simulink model "sensorExpoler_Lab_13"  (R2026a)
settings: Solver=FixedStepDiscrete  StopTime=inf  FixedStep=0.001
undefined symbols (not defined in the file): Blocking, Non
libraries: simulink x2, amg_usbconverter_n_connect_lib x2
settings Model: Creator=pboon  LastModifiedBy=Lenovo

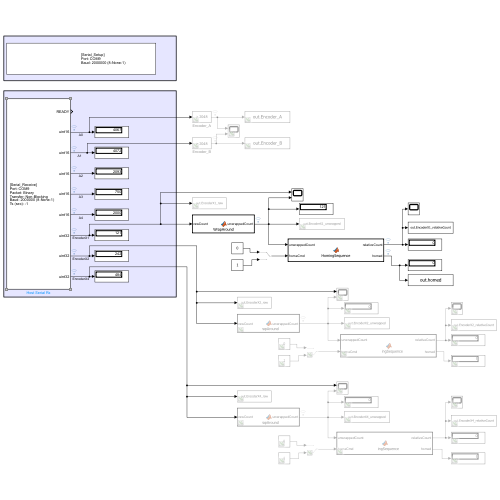
[thumbnail: Simulink's stored preview of the top-level diagram]
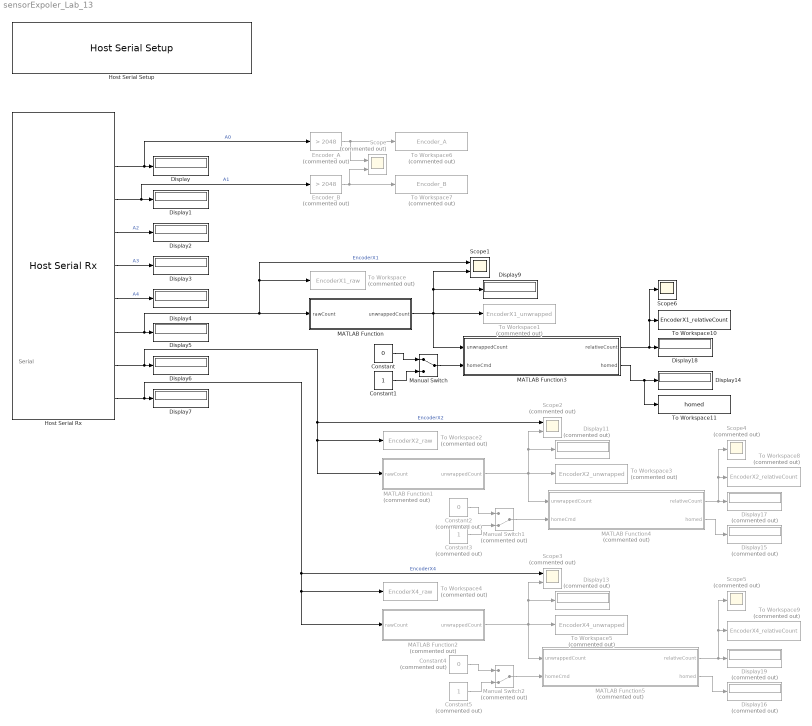
== system sensorExpoler_Lab_13 ==
  note: Serial
  Constant : Constant  Value=0
  Constant1 : Constant
  Constant2 : Constant  Commented=on  Value=0
  Constant3 : Constant  Commented=on
  Constant4 : Constant  Commented=on  Value=0
  Constant5 : Constant  Commented=on
  Display{,1..7,9,14,18} (11 alike) : Display
  Display{11,13,15..17,19} (6 alike) : Display  Commented=on
  Encoder_A : simulink/Logic and Bit Operations/Compare To Constant  Commented=on  relop=>  const=2048  OutDataTypeStr=boolean
  Encoder_B : simulink/Logic and Bit Operations/Compare To Constant  Commented=on  relop=>  const=2048  OutDataTypeStr=boolean
  Host Serial Rx : amg_usbconverter_n_connect_lib/Host Serial Rx  conf=rx  port=COM9  baudrate=2000000  databits=8  parity=None  stopbit=1  flowcontrol=None  transfer=Non-Blocking  timeout=5  packetmode=Binary  enableinitialvalues=off  initialvalues=[]  binheader='25'  binterminator='4E 4E'  porttype_double=0  porttype_single=0  porttype_int8=0  porttype_uint8=0  porttype_int16=0  porttype_uint16=5  porttype_int32=0  porttype_uint32=3  asciiformat='%d,%f'  rx_asciiterminator="CRLF (0x0D 0x0A - \"\\r\\n\")"  tx_asciiterminator="CRLF (0x0D 0x0A - \"\\r\\n\")"  sampletime=0.001  enablecustomportlabel=off  cinputportlabel=0  coutputportlabel=A  portpinstr=0  blockid=HostSerialRx  inputporttype=[]  inputportwidth=[]  inputportlabel={}  outputporttype=[3 5 5 5 5 5 7 7 7]  outputportwidth=[1 1 1 1 1 1 1 1 1]  outputportlabel={'READY','uint16','uint16','uint16','uint16','uint16','uint32','uint32','uint32'}  compat=0  optionstring=[]  autoport='COM9'
  Host Serial Setup : amg_usbconverter_n_connect_lib/Host Serial Setup  conf=setup  port=COM9  baudrate=2000000  databits=8  parity=None  stopbit=1  flowcontrol=None  transfer=Blocking  timeout=2  packetmode=Binary  initialvalues=[]  binheader='7E 7E'  binterminator='03 03'  porttype_double=0  porttype_single=1  porttype_int8=0  porttype_uint8=0  porttype_int16=0  porttype_uint16=0  porttype_int32=0  porttype_uint32=2  asciiformat='%d %u %x'  rx_asciiterminator="CRLF (0x0D 0x0A - \"\\r\\n\")"  tx_asciiterminator="CRLF (0x0D 0x0A - \"\\r\\n\")"  sampletime=-1  enablecustomportlabel=off  cinputportlabel=0  coutputportlabel=A  portpinstr=0  blockid=HostSerialSetup  inputporttype=[]  inputportwidth=[]  inputportlabel={}  outputporttype=[]  outputportwidth=[]  outputportlabel={}  compat=0  optionstring=[]  autoport='COM9'
  MATLAB Function : MATLAB Function  TreatAsAtomicUnit=on
  MATLAB Function1 : MATLAB Function  Commented=on  TreatAsAtomicUnit=on
  MATLAB Function2 : MATLAB Function  Commented=on  TreatAsAtomicUnit=on
  MATLAB Function3 : MATLAB Function  TreatAsAtomicUnit=on
  MATLAB Function4 : MATLAB Function  Commented=on  TreatAsAtomicUnit=on
  MATLAB Function5 : MATLAB Function  Commented=on  TreatAsAtomicUnit=on
  Manual Switch : ManualSwitch
  Manual Switch1 : ManualSwitch  Commented=on  CurrentSetting=0
  Manual Switch2 : ManualSwitch  Commented=on  CurrentSetting=0
  Scope : Scope  Commented=on  NumInputPorts=2
      settings: ActiveDisplayYMinimum=-0.12499999999999997  ActiveDisplayYMaximum=1.125  DataLoggingVariableName=ScopeData3
  Scope1 : Scope  NumInputPorts=2
      settings: ActiveDisplayYMinimum=-92716.012456805489  ActiveDisplayYMaximum=317138.93892092584
  Scope2 : Scope  Commented=on  NumInputPorts=2
      settings: ActiveDisplayYMinimum=-2516.4035093166231  ActiveDisplayYMaximum=6300.6367285124879
  Scope3 : Scope  Commented=on  NumInputPorts=2
      settings: ActiveDisplayYMinimum=-2516.4035093166231  ActiveDisplayYMaximum=6300.6367285124879  DataLoggingVariableName=ScopeData2
  Scope4 : Scope  Commented=on
      settings: DataLoggingVariableName=ScopeData4
  Scope5 : Scope  Commented=on
      settings: DataLoggingVariableName=ScopeData5
  Scope6 : Scope
      settings: DataLoggingVariableName=ScopeData6
  To Workspace : ToWorkspace  Commented=on  VariableName=EncoderX1_raw  SaveFormat=Timeseries  SampleTime=-1
  To Workspace1 : ToWorkspace  Commented=on  VariableName=EncoderX1_unwrapped  SaveFormat=Timeseries  SampleTime=-1
  To Workspace10 : ToWorkspace  VariableName=EncoderX1_relativeCount  SaveFormat=Timeseries  SampleTime=-1
  To Workspace11 : ToWorkspace  VariableName=homed  SaveFormat=Timeseries  SampleTime=-1
  To Workspace2 : ToWorkspace  Commented=on  VariableName=EncoderX2_raw  SaveFormat=Timeseries  SampleTime=-1
  To Workspace3 : ToWorkspace  Commented=on  VariableName=EncoderX2_unwrapped  SaveFormat=Timeseries  SampleTime=-1
  To Workspace4 : ToWorkspace  Commented=on  VariableName=EncoderX4_raw  SaveFormat=Timeseries  SampleTime=-1
  To Workspace5 : ToWorkspace  Commented=on  VariableName=EncoderX4_unwrapped  SaveFormat=Timeseries  SampleTime=-1
  To Workspace6 : ToWorkspace  Commented=on  VariableName=Encoder_A  SaveFormat=Timeseries  SampleTime=-1
  To Workspace7 : ToWorkspace  Commented=on  VariableName=Encoder_B  SaveFormat=Timeseries  SampleTime=-1
  To Workspace8 : ToWorkspace  Commented=on  VariableName=EncoderX2_relativeCount  SaveFormat=Timeseries  SampleTime=-1
  To Workspace9 : ToWorkspace  Commented=on  VariableName=EncoderX4_relativeCount  SaveFormat=Timeseries  SampleTime=-1
  wires:
  Host Serial Rx/2 -> Encoder_A/1, Display/1  "A0"
  Host Serial Rx/3 -> Encoder_B/1, Display1/1  "A1"
  Host Serial Rx/4 -> Display2/1  "A2"
  Host Serial Rx/5 -> Display3/1  "A3"
  Host Serial Rx/6 -> Display4/1  "A4"
  Host Serial Rx/7 -> To Workspace/1, Scope1/1, MATLAB Function/1(rawCount), Display5/1  "EncoderX1"
  Host Serial Rx/9 -> Scope3/1, To Workspace4/1, MATLAB Function2/1(rawCount), Display7/1  "EncoderX4"
  MATLAB Function/1(unwrappedCount) -> MATLAB Function3/1(unwrappedCount), To Workspace1/1, Scope1/2, Display9/1
  Host Serial Rx/8 -> Scope2/1, To Workspace2/1, MATLAB Function1/1(rawCount), Display6/1  "EncoderX2"
  MATLAB Function1/1(unwrappedCount) -> MATLAB Function4/1(unwrappedCount), Scope2/2, Display11/1, To Workspace3/1
  MATLAB Function2/1(unwrappedCount) -> MATLAB Function5/1(unwrappedCount), To Workspace5/1, Scope3/2, Display13/1
  Encoder_A/1 -> To Workspace6/1, Scope/1
  Encoder_B/1 -> To Workspace7/1, Scope/2
  Manual Switch/1 -> MATLAB Function3/2(homeCmd)
  Constant/1 -> Manual Switch/1
  Constant1/1 -> Manual Switch/2
  Constant2/1 -> Manual Switch1/1
  Constant3/1 -> Manual Switch1/2
  Manual Switch1/1 -> MATLAB Function4/2(homeCmd)
  Constant5/1 -> Manual Switch2/2
  Constant4/1 -> Manual Switch2/1
  Manual Switch2/1 -> MATLAB Function5/2(homeCmd)
  MATLAB Function3/2(homed) -> To Workspace11/1, Display14/1
  MATLAB Function4/2(homed) -> Display15/1
  MATLAB Function5/2(homed) -> Display16/1
  MATLAB Function4/1(relativeCount) -> Scope4/1, To Workspace8/1, Display17/1
  MATLAB Function3/1(relativeCount) -> Scope6/1, To Workspace10/1, Display18/1
  MATLAB Function5/1(relativeCount) -> Scope5/1, To Workspace9/1, Display19/1

== matlab function sensorExpoler_Lab_13/MATLAB Function ==
  data: rawCount input; unwrappedCount output
function unwrappedCount = WrapAround(rawCount)

persistent previousCount accumulatedCount initialized

MAX_COUNT  = 65535.0;
COUNT_RANGE = MAX_COUNT + 1.0;  

currentCount = double(rawCount);

if isempty(initialized)
    previousCount    = currentCount;
    accumulatedCount = 0.0;
    initialized      = true;
end

deltaCount = currentCount - previousCount;

if deltaCount < -(COUNT_RANGE / 2.0)
    deltaCount = deltaCount + COUNT_RANGE;

elseif deltaCount > (COUNT_RANGE / 2.0)
    deltaCount = deltaCount - COUNT_RANGE;
end

accumulatedCount = accumulatedCount + deltaCount;
previousCount    = currentCount;

unwrappedCount = accumulatedCount;
end

== matlab function sensorExpoler_Lab_13/MATLAB Function2 ==
  data: rawCount input; unwrappedCount output
function unwrappedCount = WrapAround(rawCount)

persistent previousCount accumulatedCount initialized

MAX_COUNT  = 65535.0;
COUNT_RANGE = MAX_COUNT + 1.0;  

currentCount = double(rawCount);

if isempty(initialized)
    previousCount    = currentCount;
    accumulatedCount = 0.0;
    initialized      = true;
end

deltaCount = currentCount - previousCount;

if deltaCount < -(COUNT_RANGE / 2.0)
    deltaCount = deltaCount + COUNT_RANGE;

elseif deltaCount > (COUNT_RANGE / 2.0)
    deltaCount = deltaCount - COUNT_RANGE;
end

accumulatedCount = accumulatedCount + deltaCount;
previousCount    = currentCount;

unwrappedCount = accumulatedCount;
end

== matlab function sensorExpoler_Lab_13/MATLAB Function3 ==
  data: unwrappedCount input; relativeCount output; homeCmd input; homed output
function [relativeCount, homed] = HomingSequence(unwrappedCount, homeCmd)

persistent homeOffset isHomed previousHomeCmd

currentCount = double(unwrappedCount);
currentHomeCmd = logical(homeCmd);

if isempty(isHomed)
    homeOffset      = 0.0;
    isHomed         = false;
    previousHomeCmd = false;
end

if currentHomeCmd && ~previousHomeCmd
    homeOffset = currentCount;
    isHomed = true;
end

if isHomed
    relativeCount = currentCount - homeOffset;
else
    relativeCount = 0.0;
end

previousHomeCmd = currentHomeCmd;
homed = double(currentHomeCmd);  

end

== matlab function sensorExpoler_Lab_13/MATLAB Function4 ==
  data: unwrappedCount input; relativeCount output; homeCmd input; homed output
function [relativeCount, homed] = HomingSequence(unwrappedCount, homeCmd)

persistent homeOffset isHomed previousHomeCmd

currentCount = double(unwrappedCount);
currentHomeCmd = logical(homeCmd);

if isempty(isHomed)
    homeOffset     = 0.0;
    isHomed        = false;
    previousHomeCmd = false;
end

if currentHomeCmd && ~previousHomeCmd
    homeOffset = currentCount;
    isHomed = true;
end

if isHomed
    relativeCount = currentCount - homeOffset;
else
    relativeCount = 0.0;
end

previousHomeCmd = currentHomeCmd;
homed = isHomed;

end

== matlab function sensorExpoler_Lab_13/MATLAB Function5 ==
  data: unwrappedCount input; relativeCount output; homeCmd input; homed output
function [relativeCount, homed] = HomingSequence(unwrappedCount, homeCmd)

persistent homeOffset isHomed previousHomeCmd

currentCount = double(unwrappedCount);
currentHomeCmd = logical(homeCmd);

if isempty(isHomed)
    homeOffset     = 0.0;
    isHomed        = false;
    previousHomeCmd = false;
end

if currentHomeCmd && ~previousHomeCmd
    homeOffset = currentCount;
    isHomed = true;
end

if isHomed
    relativeCount = currentCount - homeOffset;
else
    relativeCount = 0.0;
end

previousHomeCmd = currentHomeCmd;
homed = isHomed;

end

== matlab function sensorExpoler_Lab_13/MATLAB Function1 ==
  data: rawCount input; unwrappedCount output
function unwrappedCount = WrapAround(rawCount)

persistent previousCount accumulatedCount initialized

MAX_COUNT  = 65535.0;
COUNT_RANGE = MAX_COUNT + 1.0;  

currentCount = double(rawCount);

if isempty(initialized)
    previousCount    = currentCount;
    accumulatedCount = 0.0;
    initialized      = true;
end

deltaCount = currentCount - previousCount;

if deltaCount < -(COUNT_RANGE / 2.0)
    deltaCount = deltaCount + COUNT_RANGE;

elseif deltaCount > (COUNT_RANGE / 2.0)
    deltaCount = deltaCount - COUNT_RANGE;
end

accumulatedCount = accumulatedCount + deltaCount;
previousCount    = currentCount;

unwrappedCount = accumulatedCount;
end
